simulink model "LecBuil"  (R2020b)
settings: Solver=ode45  StartTime=0  StopTime=31449600  FixedStep=1  MaxStep=300  RelTol=1e-6
values from neighbouring files (symbols this model uses):
  P = getParameters('T_s',5,'T_s_ident',120,'Hp_val',Hp_val,'N_w',24)    [run_ident.m]    (also in run_sim.m = getParameters('T_s',5,'T_s_mpc',60))
settings Model: Creator=jpatsch  LastModifiedBy=fpaschke
settings DebuggingCC: UnderSpecifiedDimensionMsg=warning  ArithmeticOperatorsInVariantConditions=warning
settings SFSimCC: CustomCodeUndefinedFunction=UseInterfaceOnly

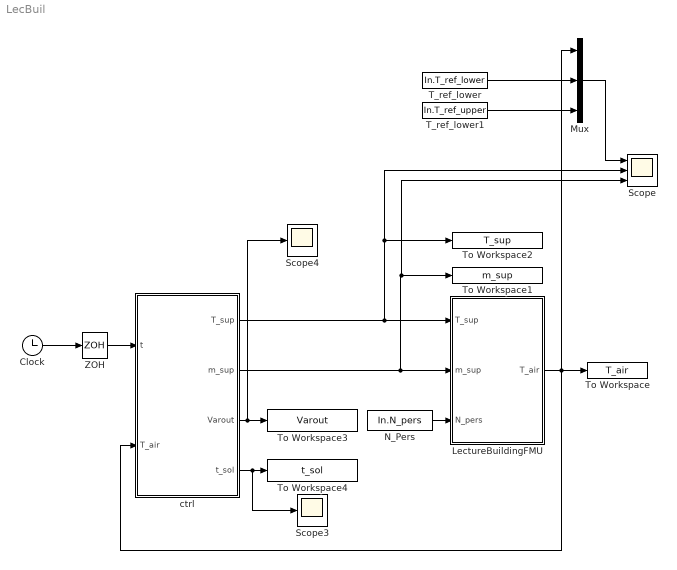
== system LecBuil ==
  Clock : Clock
  LectureBuildingFMU : Subsystem
  Mux : Mux  Inputs=3
  N_Pers : FromWorkspace  VariableName=In.N_pers  OutDataTypeStr=double  SampleTime=P.T_s*60
  Scope : Scope  NumInputPorts=3
  Scope3 : Scope
  Scope4 : Scope
  T_ref_lower : FromWorkspace  VariableName=In.T_ref_lower  OutDataTypeStr=double  SampleTime=P.T_s*60
  T_ref_lower1 : FromWorkspace  VariableName=In.T_ref_upper  OutDataTypeStr=double  SampleTime=P.T_s*60
  To Workspace : ToWorkspace  VariableName=T_air  SaveFormat=Timeseries  SampleTime=P.T_s*60
  To Workspace1 : ToWorkspace  VariableName=m_sup  SaveFormat=Timeseries  SampleTime=P.T_s*60
  To Workspace2 : ToWorkspace  VariableName=T_sup  SaveFormat=Timeseries  SampleTime=P.T_s*60
  To Workspace3 : ToWorkspace  VariableName=Varout  SaveFormat=Timeseries  SampleTime=P.T_s*60
  To Workspace4 : ToWorkspace  VariableName=t_sol  SaveFormat=Timeseries  SampleTime=P.T_s*60
  ZOH : ZeroOrderHold  SampleTime=P.T_s*60
  ctrl : MATLAB Function  TreatAsAtomicUnit=on
  wires:
  ctrl/1(T_sup) -> Scope/2, To Workspace2/1, LectureBuildingFMU/1(T_sup)
  ctrl/2(m_sup) -> Scope/3, To Workspace1/1, LectureBuildingFMU/2(m_sup)
  ZOH/1 -> ctrl/1(t)
  Clock/1 -> ZOH/1
  N_Pers/1 -> LectureBuildingFMU/3(N_pers)
  ctrl/3(Varout) -> Scope4/1, To Workspace3/1
  ctrl/4(t_sol) -> Scope3/1, To Workspace4/1
  LectureBuildingFMU/1(T_air) -> Mux/1, To Workspace/1, ctrl/2(T_air)
  T_ref_lower1/1 -> Mux/3
  T_ref_lower/1 -> Mux/2
  Mux/1 -> Scope/1

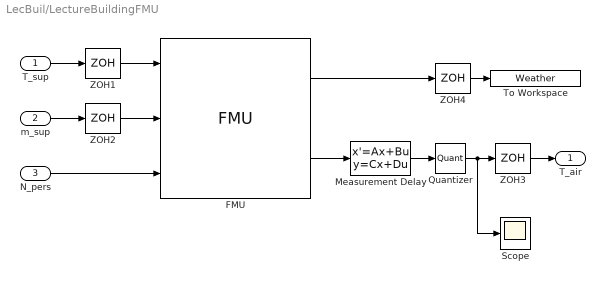
== system LecBuil/LectureBuildingFMU ==
  T_sup : Inport
  m_sup : Inport  Port=2
  N_pers : Inport  Port=3
  FMU : FMU  FMUName=LecBuilding.fmu  FMUMode=ModelExchange  h_room=[8,8,8,8,8]  l_room=[30,30,20,20,50]  w_room=[20,20,20,20,10]  h_win=[3,3,3,3,5]  w_win=[25,25,15,15,10]  Q_occ_rad=75  Q_occ_conv=25  Q_occ_lat=0  FE=struct('glass',[struct('x',0.003,'k',1.0,'tauSol',[0.834],'rhoSol_a',[0.075],'rhoSol_b',[0.075],'tauIR',0.0,'absIR_a',0.84,'absIR_b',0.84),struct('x',0.003,'k',1.0,'tauSol',[0.834],'rhoSol_a',[0.075],'rhoSol_b',[0.075],'tauIR',0.0,'absIR_a',0.84,'absIR_b',0.84)],'gas',[struct('x',0.0127,'a_k',0.002873,'b_k',7.76E-05,'a_mu',3.723E-06,'b_mu',4.94E-08,'a_c',1002.737,'b_c',0.012324,'MM',0.02897,'P0',101325.0)],'shade',struct('tauSol_a',0.1,'tauSol_b',0.1,'rhoSol_a',0.8,'rhoSol_b',0.8,'absIR_a',0.84,'absIR_b',0.84,'tauIR_a',0,'tauIR_b',0),'UFra',1.4,'absIRFra',0.8,'absSolFra',0.5)  Hs1=struct('lat',0.91664692314742,'conExtWin',[struct('glaSys',struct('haveControllableWindow',boolean(false)),'win',struct('glaUns',struct('glass',[struct('T0',293.15),struct('T0',293.15)],'gas',[struct('T0',293.15)])))],'hIntFixed',3.0,'hExtFixed',10.0,'bouConExt',struct('HDifTil',[struct('rho',0.2,'add',struct('k1',1,'k2',1)),struct('rho',0.2,'add',struct('k1',1,'k2',1))]),'bouConExtWin',struct('conPar',[struct('ove',struct('dep',0),'sidFin',struct('dep',0))],'HDifTil',[struct('rho',0.2,'add',struct('k1',1,'k2',1))],'conExtWin',[struct('radOut',struct('T0',293.15))]),'p_start',101325,'T_start',293.15,'X_start',[0.01,0.99])  Flur=struct('lat',0.91664692314742,'conExtWin',[struct('glaSys',struct('haveControllableWindow',boolean(false)),'win',struct('glaUns',struct('glass',[struct('T0',293.15),struct('T0',293.15)],'gas',[struct('T0',293.15)]))),struct('glaSys',struct('haveControllableWindow',boolean(false)),'win',struct('glaUns',struct('glass',[struct('T0',293.15),struct('T0',293.15)],'gas',[struct('T0',293.15)])))],'hIntFixed',3.0,'hExtFixed',10.0,'bouConExt',struct('HDifTil',[struct('rho',0.2,'add',struct('k1',1,'k2',1))]),'bouConExtWin',struct('conPar',[struct('ove',struct('dep',0),'sidFin',struct('dep',0)),struct('ove',struct('dep',0),'sidFin',struct('dep',0))],'HDifTil',[struct('rho',0.2,'add',struct('k1',1,'k2',1)),struct('rho',0.2,'add',struct('k1',1,'k2',1))],'conExtWin',[struct('radOut',struct('T0',293.15)),struct('radOut',struct('T0',293.15))]),'p_start',101325,'T_start',293.15,'X_start',[0.01,0.99])  Hs2=struct('lat',0.91664692314742,'conExtWin',[struct('glaSys',struct('haveControllableWindow',boolean(false)),'win',struct('glaUns',struct('glass',[struct('T0',293.15),struct('T0',293.15)],'gas',[struct('T0',293.15)])))],'hIntFixed',3.0,'hExtFixed',10.0,'bouConExt',struct('HDifTil',[struct('rho',0.2,'add',struct('k1',1,'k2',1)),struct('rho',0.2,'add',struct('k1',1,'k2',1))]),'bouConExtWin',struct('conPar',[struct('ove',struct('dep',0),'sidFin',struct('dep',0))],'HDifTil',[struct('rho',0.2,'add',struct('k1',1,'k2',1))],'conExtWin',[struct('radOut',struct('T0',293.15))]),'p_start',101325,'T_start',293.15,'X_start',[0.01,0.99])  Hs3=struct('lat',0.91664692314742,'conExtWin',[struct('glaSys',struct('haveControllableWindow',boolean(false)),'win',struct('glaUns',struct('glass',[struct('T0',293.15),struct('T0',293.15)],'gas',[struct('T0',293.15)])))],'hIntFixed',3.0,'hExtFixed',10.0,'bouConExt',struct('HDifTil',[struct('rho',0.2,'add',struct('k1',1,'k2',1)),struct('rho',0.2,'add',struct('k1',1,'k2',1))]),'bouConExtWin',struct('conPar',[struct('ove',struct('dep',0),'sidFin',struct('dep',0))],'HDifTil',[struct('rho',0.2,'add',struct('k1',1,'k2',1))],'conExtWin',[struct('radOut',struct('T0',293.15))]),'p_start',101325,'T_start',293.15,'X_start',[0.01,0.99])  Hs4=struct('lat',0.91664692314742,'conExtWin',[struct('glaSys',struct('haveControllableWindow',boolean(false)),'win',struct('glaUns',struct('glass',[struct('T0',293.15),struct('T0',293.15)],'gas',[struct('T0',293.15)])))],'hIntFixed',3.0,'hExtFixed',10.0,'bouConExt',struct('HDifTil',[struct('rho',0.2,'add',struct('k1',1,'k2',1)),struct('rho',0.2,'add',struct('k1',1,'k2',1))]),'bouConExtWin',struct('conPar',[struct('ove',struct('dep',0),'sidFin',struct('dep',0))],'HDifTil',[struct('rho',0.2,'add',struct('k1',1,'k2',1))],'conExtWin',[struct('radOut',struct('T0',293.15))]),'p_start',101325,'T_start',293.15,'X_start',[0.01,0.99])  weaDat=struct('pAtm',101325,'TDryBul',293.15,'TDewPoi',283.15,'TBlaSky',273.15,'relHum',0.5,'winSpe',1,'winDir',1.0,'HInfHor',0.0,'ceiHei',20000,'totSkyCov',0.5,'opaSkyCov',0.5)  Zul1=struct('X_2',[0.01,0.99],'m_flow',2,'T',293.15)  Zul2=struct('X_2',[0.01,0.99],'m_flow',2,'T',293.15)  Zul3=struct('X_2',[0.01,0.99],'m_flow',1.5,'T',293.15)  Zul4=struct('X_2',[0.01,0.99],'m_flow',1.5,'T',293.15)  T_ZulToK=struct('k1',1,'k2',1)  FB=struct('absIR_a',0.9,'absIR_b',0.9,'absSol_a',0.5,'absSol_b',0.5,'roughness_a',int32(3))  IW=struct('absIR_a',0.9,'absIR_b',0.9,'absSol_a',0.5,'absSol_b',0.5,'roughness_a',int32(3))  BodenPlatte=struct('T_a_start',293.15,'T_b_start',293.15)  bouPres=struct('X_2',[0.01,0.99],'p',100000,'T',293.15)  AW=struct('absIR_a',0.9,'absIR_b',0.9,'absSol_a',0.5,'absSol_b',0.5,'roughness_a',int32(3))  gai1=struct('K_2',reshape([0,0,0], [3,1]))  mask(LecBuilding [Model Exchange, v2.0]){}
      settings: MultiThreadCoSim=off
      mask Display:
      | disp('LecBuilding');
      | port_label('output',1,'weaBus');
      | port_label('output',2,'T_air');
      | port_label('input',1,'T_Sup');
      | port_label('input',2,'M_Sup');
      | port_label('input',3,'N_Pers');
  Measurement Delay : StateSpace  A=-eye(5)./(P.T_sens*60)  B=eye(5)./(P.T_sens*60)  C=eye(5)  D=zeros(5)  InitialCondition=20*ones(5,1)
  Quantizer : Quantizer  QuantizationInterval=P.Q_int
  Scope : Scope
  To Workspace : ToWorkspace  VariableName=Weather  SaveFormat=Timeseries  SampleTime=P.T_s*60
  ZOH{1..4} (4 alike) : ZeroOrderHold  SampleTime=P.T_s*60
  T_air : Outport
  wires:
  Measurement Delay/1 -> Quantizer/1
  T_sup/1 -> ZOH1/1
  Quantizer/1 -> Scope/1, ZOH3/1
  ZOH1/1 -> FMU/1
  ZOH2/1 -> FMU/2
  N_pers/1 -> FMU/3
  ZOH3/1 -> T_air/1
  m_sup/1 -> ZOH2/1
  FMU/2 -> Measurement Delay/1
  FMU/1 -> ZOH4/1
  ZOH4/1 -> To Workspace/1

== matlab function LecBuil/ctrl ==
  data: t input size=1; T_air input size=5; T_sup output size=1; m_sup output size=4; Varout output size=4; t_sol output
function [T_sup, m_sup, Varout, t_sol] = ctrl(t,T_air)
%Calls controller function.
%
% [T_sup, m_sup, T_air_obs, t_sol] = ctrl(t,T_air)

T_sup = NaN;
m_sup = NaN(4,1);
Varout = NaN(4,1);
t_sol = NaN;
coder.extrinsic('ctrl_fun');
[T_sup, m_sup, Varout, t_sol] = ctrl_fun(t,T_air);
end
